simulink model "Simple_caps_working4"  (R2018b)
settings: Solver=ode5  StartTime=0.0  StopTime=10  FixedStep=Ts  RelTol=1e-3
PreLoadFcn:
  | setMatlabPaths
  | Ts = 1e-4
  | C = 100e-6
undefined symbols (not defined in the file or in its folder): DiscIntNeverNeededParam, sigbuilder_block
libraries: Simple_lib x61, peGeneralControl x3, simulink x1
settings Model: NumberOfSteps=1000  Creator=billw  LastModifiedBy=billw

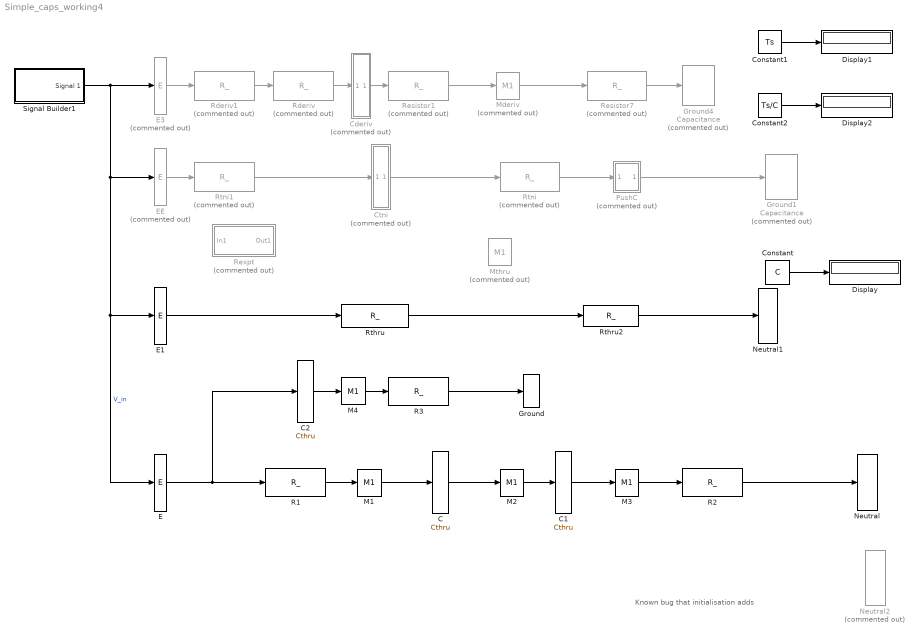
== system Simple_caps_working4 ==
  note: Known bug that initialisation adds
  C : Simple_lib/Electronics/Cthru  C=C  Q_0=0
      settings: AttributesFormatString=%<C>F
  C1 : Simple_lib/Electronics/Cthru  C=C  Q_0=0
      settings: AttributesFormatString=%<C>F
  C2 : Simple_lib/Electronics/Cthru  C=0.001  Q_0=0
      settings: AttributesFormatString=%<C>F
  "Cderiv " : Subsystem  Commented=on  mask{C=C, Q_0=0}
      mask prompts: C "Capacitance"; Q_0 "Initial Charge (C)"
      settings: AttributesFormatString=%<C>F
      mask Display:
      | %plot([1.0 1.8 1.8 1.0], [0 .1 -.1 0])
      | %patch([-1 -1 -.7 -.7 -1], [-1 1 1 -1 -1])
      | %patch([1 1 .7 .7 1], [-1 1 1 -1 -1])
      | plot([-1 -1], [-1 1])
      | plot([1 1], [-1 1])
      | color('white')
      | plot([-1.1 -1.1], [-1 1])
      | plot([1.1 1.1], [-1 1])
  Constant : Constant  Value=C
  Constant1 : Constant  Value=Ts
  Constant2 : Constant  Value=Ts/C
  Ctni : Subsystem  Commented=on  mask{C=C, Q_0=0}
      mask prompts: C "Capacitance"; Q_0 "Initial Charge (C)"
      settings: AttributesFormatString=%<C>F
      mask Display:
      | %plot([1.0 1.8 1.8 1.0], [0 .1 -.1 0])
      | %patch([-1 -1 -.7 -.7 -1], [-1 1 1 -1 -1])
      | %patch([1 1 .7 .7 1], [-1 1 1 -1 -1])
      | plot([-1 -1], [-1 1])
      | plot([1 1], [-1 1])
      | color('white')
      | plot([-1.1 -1.1], [-1 1])
      | plot([1.1 1.1], [-1 1])
  Display : Display
  Display1 : Display
  Display2 : Display
  E : Simple_lib/Electronics/E  Vbatt=0
      settings: AttributesFormatString=EMF: %<Vbatt> V
  E1 : Simple_lib/Electronics/E  Vbatt=0
      settings: AttributesFormatString=EMF: %<Vbatt> V
  E3 : Simple_lib/Electronics/E  Commented=on  Vbatt=0
      settings: AttributesFormatString=EMF: %<Vbatt> V
  EE : Simple_lib/Electronics/E  Commented=on  Vbatt=0
      settings: AttributesFormatString=EMF: %<Vbatt> V
  Ground : Simple_lib/Electronics/Ground  SystemSampleTime=-1
      link override Rgnd: R=1
  Ground1 : Simple_lib/Electronics/Capacitance  Commented=on  C=inf  V0=0
      settings: AttributesFormatString=%<C> F
  Ground4 : Simple_lib/Electronics/Capacitance  Commented=on  C=inf  V0=0
      settings: AttributesFormatString=%<C> F
  M{1..4} (4 alike) : Simple_lib/Electronics/M1  SystemSampleTime=-1
  Mderiv : Simple_lib/Electronics/M1  Commented=on  SystemSampleTime=-1
  Mthru : Simple_lib/Electronics/M1  Commented=on  SystemSampleTime=-1
  Neutral : Simple_lib/Electronics/Neutral  V0=0
      settings: AttributesFormatString=%<V0> V
  Neutral1 : Simple_lib/Electronics/Neutral  V0=-10
      settings: AttributesFormatString=%<V0> V
  Neutral2 : Simple_lib/Electronics/Neutral  Commented=on  V0=-9
      settings: AttributesFormatString=%<V0> V
  PushC : Subsystem  Commented=on  mask{C=C}
      mask prompts: C "Capacitance (Farads)"
      mask Display:
      | plot([-1 -.9 -.5 0 .5 .9 1  .9  .5  0 -.5 -.9 -1],      [ 0  .5 .9 1 .9 .5 0 -.5 -.9 -1 -.9 -.5  0]);
      | disp('M')
  R1 : Simple_lib/Electronics/R_  Exponent=3  R=1000
      settings: AttributesFormatString=%<R> Ohm
  R2 : Simple_lib/Electronics/R_  Exponent=3  R=1000
      link override at: slew_rate=inf
      settings: AttributesFormatString=%<R> Ohm
  R3 : Simple_lib/Electronics/R_  Exponent=3  R=1000
      settings: AttributesFormatString=%<R> Ohm
  Rderiv : Simple_lib/Electronics/R_  Commented=on  Exponent=0  R=1
      settings: AttributesFormatString=%<R> Ohm
  Rderiv1 : Simple_lib/Electronics/R_  Commented=on  Exponent=0  R=1
      settings: AttributesFormatString=%<R> Ohm
  Resistor1 : Simple_lib/Electronics/R_  Commented=on  Exponent=0  R=1
      link override at: slew_rate=inf
      link override at/Saturation1: LowerLimit=1e-24
      link override thru/1//R1: Gain=-1
      settings: AttributesFormatString=%<R> Ohm
  Resistor7 : Simple_lib/Electronics/R_  Commented=on  Exponent=0  R=1
      link override at: slew_rate=inf
      link override at/Saturation1: LowerLimit=1e-24
      link override thru/1//R1: Gain=-1
      settings: AttributesFormatString=%<R> Ohm
  Rexpt : Subsystem  Commented=on  AncestorBlock=Simple_lib/Electronics/R_  mask(Circuit Resistor){Mantissa=1.0, Exponent=0, R=1}
      mask prompts: Mantissa "Resistance (Ohm)"; Exponent "e"
      mask help: This block contains an Ohmic Resistance, and a test point at its outport.
      mask init:
      | newR = str2num(Mantissa) * 10^Exponent;
      | set(gcbh,'R', num2str(newR))
      settings: AttributesFormatString=%<R> Ohm
      mask Help:
      | Choose one of the standard resistance values or type your own.
      | e means the power of 10 that the chosen resistance value will be multiplied by to make the actual resistance used.
      mask TypeOptions Mantissa: 1.0 | 1.2 | 1.5 | 1.8 | 2.2 | 2.7 | 3.3 | 3.9 | 4.7 | 5.6 | 6.8 | 8.2
      mask DialogControl Exponent Tooltip: Times this power of ten
      mask Display:
      | %color('black')
      | %plot([1.0 1.18 1.18 1.0], [0 .2 -.2 0])
      | plot([-8:8]/8, [0 1 0 -1 0 1 0 -1 0 1 0 -1 0 1 0 -1 0])
      | 
      | color('white')
      | plot([-1 1 1 -1 -1], [-1 -1 1 1 -1])
  Rthru : Simple_lib/Electronics/R_  Exponent=3  R=1000
      settings: AttributesFormatString=%<R> Ohm
  Rthru2 : Simple_lib/Electronics/R_  Exponent=3  R=1000
      settings: AttributesFormatString=%<R> Ohm
  Rtni : Simple_lib/Electronics/R_  Commented=on  Exponent=0  R=1
      settings: AttributesFormatString=%<R> Ohm
  Rtni1 : Simple_lib/Electronics/R_  Commented=on  Exponent=0  R=1
      settings: AttributesFormatString=%<R> Ohm
  Signal Builder1 : Subsystem  Tag=STV Subsys  LoadFcn=sigbuilder_block('load');  StartFcn=sigbuilder_block('start');  StopFcn=sigbuilder_block('stop');  ClipboardFcn=sigbuilder_block('clipboard');  mask(Sigbuilder block){tuvar=[0:10]}
      mask help: Simulink:masks:SigbuilderBlock_MD
      mask init:
      | if ~strcmp(get_param(bdroot(gcbh),'SimulationStatus'),'stopped') tuvar = sigbuilder_block('maskInit'); end
      settings: CopyFcn=sigbuilder_block('copy');  DeleteFcn=sigbuilder_block('delete');  ModelCloseFcn=sigbuilder_block('modelClose');  PreSaveFcn=sigbuilder_block('preSave');  PauseFcn=sigbuilder_block('pause');  ContinueFcn=sigbuilder_block('continue');  NameChangeFcn=sigbuilder_block('namechange');  OpenFcn=sigbuilder_block('open',[601.8 232.8 544.8 353.4 ]);  CloseFcn=sigbuilder_block('close');
      mask Display: plot(0, 0, 100, 100,[2, 2, 32, 32, 2], [68, 8, 8, 68, 68],[32, 2], [38, 38], [32, 19, 2],[53, 60, 44], [32, 17, 17, 2],[16, 16, 31, 31]);txt = getActiveGroup(gcbh);text(2, 100, txt,'verticalAlignment', 'top');
  wires:
  PushC/1(Out1) -> Ground1/1
  EE/1 -> Rtni1/1
  Rtni/1 -> PushC/1(In1)
  Mderiv/1 -> Resistor7/1
  E3/1 -> Rderiv1/1
  Rderiv/1 -> "Cderiv "/1(In1)
  "Cderiv "/1(Out1) -> Resistor1/1
  E1/1 -> Rthru/1
  Rthru/1 -> Rthru2/1
  Resistor1/1 -> Mderiv/1
  Resistor7/1 -> Ground4/1
  Rtni1/1 -> Ctni/1(In1)
  Rderiv1/1 -> Rderiv/1
  Ctni/1(Out1) -> Rtni/1
  Constant/1 -> Display/1
  Constant2/1 -> Display2/1
  Constant1/1 -> Display1/1
  Rthru2/1 -> Neutral1/1
  Signal Builder1/1(Signal 1) -> E/1, E1/1, EE/1, E3/1  "V_in"
  R1/1 -> M1/1
  M1/1 -> C/1
  E/1 -> C2/1, R1/1
  C/1 -> M2/1
  M2/1 -> C1/1
  R2/1 -> Neutral/1
  C1/1 -> M3/1
  M3/1 -> R2/1
  C2/1 -> M4/1
  R3/1 -> Ground/1
  M4/1 -> R3/1

== system Simple_caps_working4/Cderiv  ==
  In1 : Inport
  C2 : Subsystem  Commented=on  AncestorBlock=Simple_lib/Electronics/C1  mask{C=1e-3}
      mask prompts: C "Capacitance"
      settings: AttributesFormatString=%<C> F
      mask Display:
      | plot([-1 1], [0.5 0.5])
      | plot([-1 1], [-0.5 -0.5])
      | 
      | 
      | color('white')
      | plot([-1 1 1 -1 -1], [-1 -1 1 1 -1])
  C3 : Subsystem  AncestorBlock=Simple_lib/Electronics/C1  mask{C=1e-3}
      mask prompts: C "Capacitance"
      settings: AttributesFormatString=%<C> F
      mask Display:
      | plot([-1 1], [0.5 0.5])
      | plot([-1 1], [-0.5 -0.5])
      | 
      | 
      | color('white')
      | plot([-1 1 1 -1 -1], [-1 -1 1 1 -1])
  Cap : Subsystem  Commented=on  AncestorBlock=Simple_lib/Electronics/C1  mask{C=C}
      mask prompts: C "Capacitance"
      settings: AttributesFormatString=%<C> F
      mask Display:
      | plot([-1 1], [0.5 0.5])
      | plot([-1 1], [-0.5 -0.5])
      | 
      | 
      | color('white')
      | plot([-1 1 1 -1 -1], [-1 -1 1 1 -1])
  Cgood : Subsystem  AncestorBlock=Simple_lib/Electronics/C1  mask{C=10e-6}
      mask prompts: C "Capacitance"
      settings: AttributesFormatString=%<C> F
      mask Display:
      | plot([-1 1], [0.5 0.5])
      | plot([-1 1], [-0.5 -0.5])
      | 
      | 
      | color('white')
      | plot([-1 1 1 -1 -1], [-1 -1 1 1 -1])
  from : Simple_lib/Electronics/TP  V_0=0.0  C=0  conserved_quantity_name=Q  energy_name=E
  Out1 : Outport
  wires:
  In1/1 -> C3/2(neg)
  from/1 -> C3/1(pos), Out1/1

== system Simple_caps_working4/Ctni ==
  In1 : Inport
  C2 : Subsystem  Commented=on  AncestorBlock=Simple_lib/Electronics/C1  mask{C=1e-3}
      mask prompts: C "Capacitance"
      settings: AttributesFormatString=%<C> F
      mask Display:
      | plot([-1 1], [0.5 0.5])
      | plot([-1 1], [-0.5 -0.5])
      | 
      | 
      | color('white')
      | plot([-1 1 1 -1 -1], [-1 -1 1 1 -1])
  C3 : Subsystem  AncestorBlock=Simple_lib/Electronics/C1  mask{C=1e-3}
      mask prompts: C "Capacitance"
      settings: AttributesFormatString=%<C> F
      mask Display:
      | plot([-1 1], [0.5 0.5])
      | plot([-1 1], [-0.5 -0.5])
      | 
      | 
      | color('white')
      | plot([-1 1 1 -1 -1], [-1 -1 1 1 -1])
  Cap : Subsystem  Commented=on  AncestorBlock=Simple_lib/Electronics/C1  mask{C=C}
      mask prompts: C "Capacitance"
      settings: AttributesFormatString=%<C> F
      mask Display:
      | plot([-1 1], [0.5 0.5])
      | plot([-1 1], [-0.5 -0.5])
      | 
      | 
      | color('white')
      | plot([-1 1 1 -1 -1], [-1 -1 1 1 -1])
  Cgood : Subsystem  AncestorBlock=Simple_lib/Electronics/C1  mask{C=10e-6}
      mask prompts: C "Capacitance"
      settings: AttributesFormatString=%<C> F
      mask Display:
      | plot([-1 1], [0.5 0.5])
      | plot([-1 1], [-0.5 -0.5])
      | 
      | 
      | color('white')
      | plot([-1 1 1 -1 -1], [-1 -1 1 1 -1])
  from : Simple_lib/Electronics/TP  V_0=0.0  C=0  conserved_quantity_name=Q  energy_name=E
  Out1 : Outport
  wires:
  In1/1 -> C3/2(neg)
  from/1 -> C3/1(pos), Out1/1

== system Simple_caps_working4/PushC ==
  In1 : Inport
  SeriesCapacitance : Subsystem
  _at : Simple_lib/Electronics/_out  Tag=Electrical  Level=V  Flow=I
  _thru : Subsystem  AncestorBlock=Simple_lib/Electronics/_in  InitFcn=""  mask{Level=V, Flow=I}
      mask prompts: Level "Level variable name:"; Flow "Flow variable name:"
      mask init:
      | init_in
      mask Display:
      | %% Icon for flow in
      | % Signally design
      | %plot([0 2 2 3], [1 1 0 0])
      | %plot([1 3 2 1 0 2], [0.6 0.6 0.4 0.6 0.4 0.4])
      | %patch([1 3 2],[0.6 0.6 0.4])
      | %plot([0 1 1], [1 1 0.6])
      | %plot([1 1 0], [0.4 -1 -1])
      | 
      | %color('white')
      | %plot([0 3], [2 2])
      | %plot([0 3], [-2 -2])
      | 
      | %% Bolder design
      | %patch( [0 1 -1], [0 1 1])
      | %plot( [-1 1], [1.05 1.05])
      | %patch( [-0.1 -0.1 -1], [0.95 0 0.95])
      | patch( [-0.1 -0.1 -1], [1 0 1])
      | patch( [0.1 0.1 1], [1 0 1])
      | plot( [0.1 1 -1 -0.1], [0 -2 -2 0]*0.5)
      | %patch( [-0.1 0.1 0.1 -0.1], [0 0 1 1], [1 1 1])
      | %patch( [-1 0.1 0.1 -1], [1 1 0.95 0.95], [1 1 1])
      | 
      | %% Size the box
      | color('white')
      | plot( [-1 1], [2 2])
      | plot( [-1 1], -[2 2])
  Out1 : Outport
  wires:
  In1/1 -> _thru/1(in)
  _at/1 -> Out1/1
  _thru/1(out) -> _at/1
  _at/2 -> SeriesCapacitance/1(In1)
  SeriesCapacitance/1(Out1) -> _thru/2(back)

== system Simple_caps_working4/Rexpt ==
  In1 : Inport
  Math Function : Math  Operator=reciprocal  SaturateOnIntegerOverflow=on
  R1 : Simple_lib/Electronics/R1  Commented=on  R=R
      settings: AttributesFormatString=%<R> Ohms
  Sine Wave : Sin  Amplitude=.1  Bias=.2  SampleTime=0
  VR : Simple_lib/Electronics/VR  SystemSampleTime=-1
  at : Subsystem  AncestorBlock=Simple_lib/Electronics/TP  mask{V_0=20, slew_rate=1000, conserved_quantity_name=Q, energy_name=E}
      mask prompts: V_0 "Iniitial Potential (V)"; slew_rate "Max +/- slew rate (V/s)"; conserved_quantity_name "Conserved quantity name"; energy_name "Energy name"
      mask init:
      | init_lump
      mask Display:
      | plot([-1 -.9 -.5 0 .5 .9 1  .9  .5  0 -.5 -.9 -1],      [ 0  .5 .9 1 .9 .5 0 -.5 -.9 -1 -.9 -.5  0]);
      | %disp(get(gcbh,'Name'))
  Out1 : Outport
  wires:
  at/1(out) -> VR/3, Out1/1
  In1/1 -> VR/1
  Sine Wave/1 -> Math Function/1  "R"
  Math Function/1 -> VR/2  "G"

== system Simple_caps_working4/Signal Builder1 ==
  Demux : Demux  Tag=STV Demux  Outputs=1
  FromWs : FromWorkspace  Tag=STV FromWs  VariableName=tuvar  SampleTime=0
      SigBuilderData=|
      | common.afterFinalStr = 'Extrapolate'
      | common.sampleTime = 0
      | dataSet.timeRange = [0 10]
      | dataSet.name = 'Group 1'
      | sbobj.Groups.Name = 'Group 1'
      | sbobj.Groups.Signals.Name = 'Signal 1'
      | sbobj.Groups.Signals.XData = [0 2.98 2.98 4 4 6 6 10]
      | sbobj.Groups.Signals.YData = [0.39 0.39 0.5 0.5 1 1 0.225 0.225]
  Signal 1 : Outport  Tag=STV Outport
  wires:
  FromWs/1 -> Demux/1
  Demux/1 -> Signal 1/1

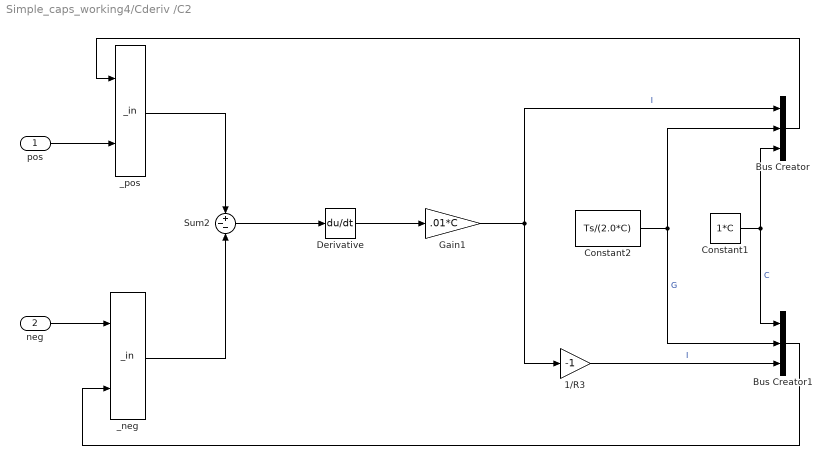
== system Simple_caps_working4/Cderiv /C2 ==
  pos : Inport
  neg : Inport  Port=2
  1/R3 : Gain  Gain=-1
  Bus Creator : BusCreator  Inputs=3
  Bus Creator1 : BusCreator  Inputs=3
  Constant1 : Constant  Value=1*C
  Constant2 : Constant  Value=Ts/(2.0*C)
  Derivative : Derivative
  Gain1 : Gain  Gain=.01*C
  Sum2 : Sum  Inputs=+--
  _neg : Simple_lib/Electronics/_in  Level=V  Flow=I
  _pos : Simple_lib/Electronics/_in  Level=V  Flow=I
  wires:
  Constant1/1 -> Bus Creator/3, Bus Creator1/1  "C"
  Constant2/1 -> Bus Creator/2, Bus Creator1/2  "G"
  1/R3/1 -> Bus Creator1/3  "I"
  Sum2/1 -> Derivative/1
  _neg/1 -> Sum2/3
  Bus Creator1/1 -> _neg/2
  Bus Creator/1 -> _pos/2
  _pos/1 -> Sum2/1
  pos/1 -> _pos/1
  neg/1 -> _neg/1
  Derivative/1 -> Gain1/1
  Gain1/1 -> 1/R3/1, Bus Creator/1  "I"

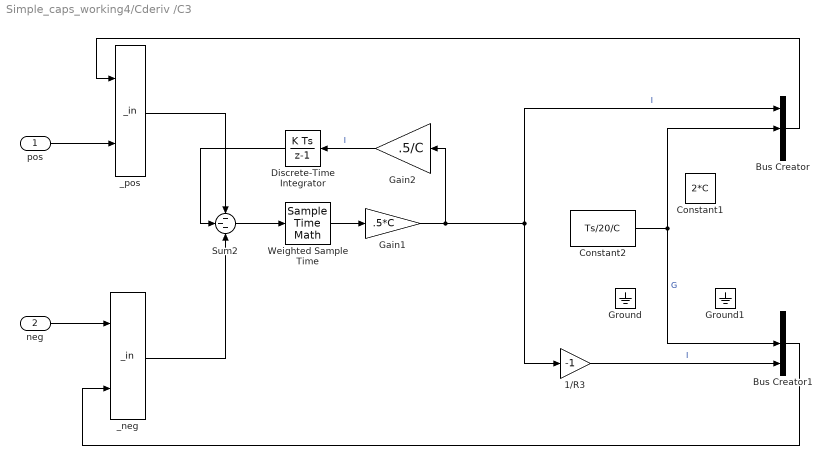
== system Simple_caps_working4/Cderiv /C3 ==
  pos : Inport
  neg : Inport  Port=2
  1/R3 : Gain  Gain=-1
  Bus Creator : BusCreator  Inputs=3
  Bus Creator1 : BusCreator  Inputs=3
  Constant1 : Constant  Value=2*C
  Constant2 : Constant  Value=Ts/20/C
  Discrete-Time Integrator : DiscreteIntegrator  SampleTime=-1  ICPrevOutput=DiscIntNeverNeededParam  ICPrevScaledInput=DiscIntNeverNeededParam
  Gain1 : Gain  Gain=.5*C
  Gain2 : Gain  Gain=.5/C
  Ground : Ground
  Ground1 : Ground
  Sum2 : Sum  Inputs=---
  Weighted Sample Time : SampleTimeMath  TsampMathOp=/  weightValue=1.1
  _neg : Simple_lib/Electronics/_in  Level=V  Flow=I
  _pos : Simple_lib/Electronics/_in  Level=V  Flow=I
  wires:
  ? -> Bus Creator/3, Bus Creator1/1  "C"
  Constant2/1 -> Bus Creator/2, Bus Creator1/2  "G"
  1/R3/1 -> Bus Creator1/3  "I"
  Sum2/1 -> Weighted Sample Time/1
  _neg/1 -> Sum2/3
  Bus Creator1/1 -> _neg/2
  Bus Creator/1 -> _pos/2
  _pos/1 -> Sum2/1
  pos/1 -> _pos/1
  neg/1 -> _neg/1
  Weighted Sample Time/1 -> Gain1/1
  Gain1/1 -> 1/R3/1, Bus Creator/1, Gain2/1  "I"
  Discrete-Time Integrator/1 -> Sum2/2
  Gain2/1 -> Discrete-Time Integrator/1  "I"

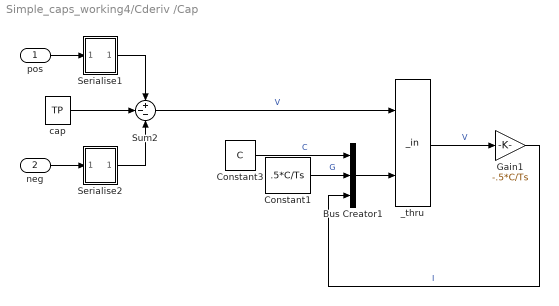
== system Simple_caps_working4/Cderiv /Cap ==
  pos : Inport
  neg : Inport  Port=2
  Bus Creator1 : BusCreator  Inputs=3
  Constant1 : Constant  Value=.5*C/Ts
  Constant3 : Constant  Value=C
  Gain1 : Gain  Gain=-.5*C/Ts
  Serialise1 : Subsystem
      mask Display:
      | plot([-1 -.9 -.5 0 .5 .9 1  .9  .5  0 -.5 -.9 -1],      [ 0  .5 .9 1 .9 .5 0 -.5 -.9 -1 -.9 -.5  0]);
      | disp('M')
  Serialise2 : Subsystem
      mask Display:
      | plot([-1 -.9 -.5 0 .5 .9 1  .9  .5  0 -.5 -.9 -1],      [ 0  .5 .9 1 .9 .5 0 -.5 -.9 -1 -.9 -.5  0]);
      | disp('M')
  Sum2 : Sum  Inputs=+--
  _thru : Simple_lib/Electronics/_in  Level=V  Flow=I
  cap : Simple_lib/Electronics/TP  V_0=0.0  C=0  conserved_quantity_name=Q  energy_name=E
      link override Saturation1: LowerLimit=0
  wires:
  pos/1 -> Serialise1/1(In1)
  Bus Creator1/1 -> _thru/2
  neg/1 -> Serialise2/1(In1)
  Constant1/1 -> Bus Creator1/2  "G"
  Constant3/1 -> Bus Creator1/1  "C"
  Gain1/1 -> Bus Creator1/3  "I"
  _thru/1 -> Gain1/1  "V"
  Sum2/1 -> _thru/1  "V"
  Serialise1/1(Out1) -> Sum2/1
  Serialise2/1(Out1) -> Sum2/3
  cap/1 -> Sum2/2

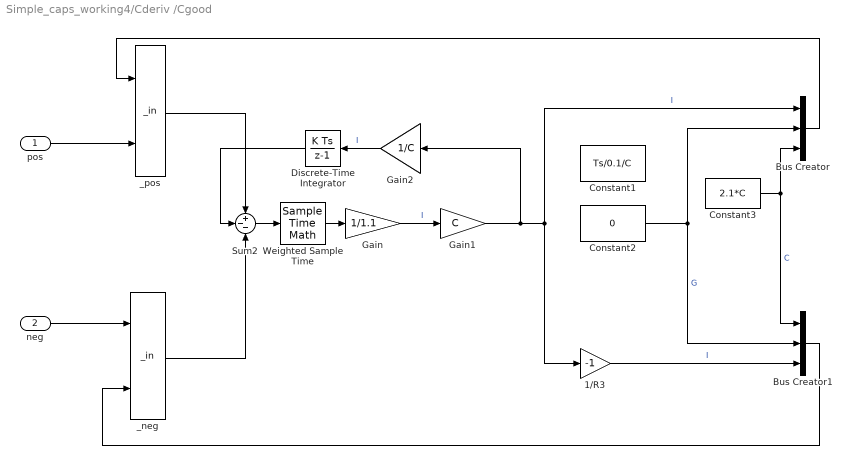
== system Simple_caps_working4/Cderiv /Cgood ==
  pos : Inport
  neg : Inport  Port=2
  1/R3 : Gain  Gain=-1
  Bus Creator : BusCreator  Inputs=3
  Bus Creator1 : BusCreator  Inputs=3
  Constant1 : Constant  Value=Ts/0.1/C
  Constant2 : Constant  Value=0
  Constant3 : Constant  Value=2.1*C
  Discrete-Time Integrator : DiscreteIntegrator  SampleTime=-1  ICPrevOutput=DiscIntNeverNeededParam  ICPrevScaledInput=DiscIntNeverNeededParam
  Gain : Gain  Gain=1/1.1
  Gain1 : Gain  Gain=C
  Gain2 : Gain  Gain=1/C
  Sum2 : Sum  Inputs=+--
  Weighted Sample Time : SampleTimeMath  TsampMathOp=/  weightValue=1
  _neg : Simple_lib/Electronics/_in  Level=V  Flow=I
  _pos : Simple_lib/Electronics/_in  Level=V  Flow=I
  wires:
  Gain2/1 -> Discrete-Time Integrator/1  "I"
  Discrete-Time Integrator/1 -> Sum2/2
  Gain/1 -> Gain1/1  "I"
  Weighted Sample Time/1 -> Gain/1
  _pos/1 -> Sum2/1
  Bus Creator/1 -> _pos/2
  Bus Creator1/1 -> _neg/2
  _neg/1 -> Sum2/3
  Sum2/1 -> Weighted Sample Time/1
  1/R3/1 -> Bus Creator1/3  "I"
  Constant2/1 -> Bus Creator1/2, Bus Creator/2  "G"
  Constant3/1 -> Bus Creator1/1, Bus Creator/3  "C"
  pos/1 -> _pos/1
  neg/1 -> _neg/1
  Gain1/1 -> Gain2/1, Bus Creator/1, 1/R3/1  "I"

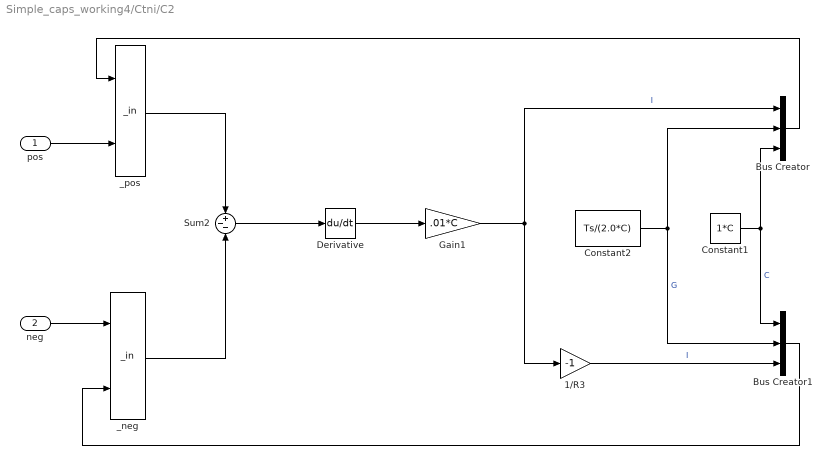
== system Simple_caps_working4/Ctni/C2 ==
  pos : Inport
  neg : Inport  Port=2
  1/R3 : Gain  Gain=-1
  Bus Creator : BusCreator  Inputs=3
  Bus Creator1 : BusCreator  Inputs=3
  Constant1 : Constant  Value=1*C
  Constant2 : Constant  Value=Ts/(2.0*C)
  Derivative : Derivative
  Gain1 : Gain  Gain=.01*C
  Sum2 : Sum  Inputs=+--
  _neg : Simple_lib/Electronics/_in  Level=V  Flow=I
  _pos : Simple_lib/Electronics/_in  Level=V  Flow=I
  wires:
  Constant1/1 -> Bus Creator/3, Bus Creator1/1  "C"
  Constant2/1 -> Bus Creator/2, Bus Creator1/2  "G"
  1/R3/1 -> Bus Creator1/3  "I"
  Sum2/1 -> Derivative/1
  _neg/1 -> Sum2/3
  Bus Creator1/1 -> _neg/2
  Bus Creator/1 -> _pos/2
  _pos/1 -> Sum2/1
  pos/1 -> _pos/1
  neg/1 -> _neg/1
  Derivative/1 -> Gain1/1
  Gain1/1 -> 1/R3/1, Bus Creator/1  "I"

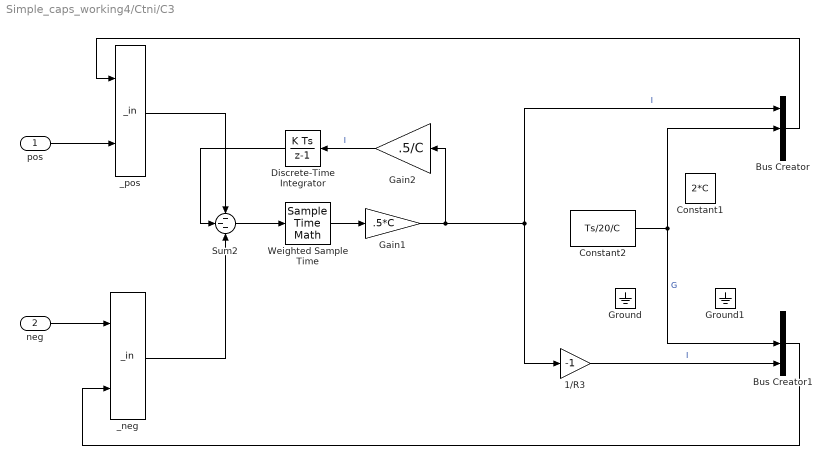
== system Simple_caps_working4/Ctni/C3 ==
  pos : Inport
  neg : Inport  Port=2
  1/R3 : Gain  Gain=-1
  Bus Creator : BusCreator  Inputs=3
  Bus Creator1 : BusCreator  Inputs=3
  Constant1 : Constant  Value=2*C
  Constant2 : Constant  Value=Ts/20/C
  Discrete-Time Integrator : DiscreteIntegrator  SampleTime=-1  ICPrevOutput=DiscIntNeverNeededParam  ICPrevScaledInput=DiscIntNeverNeededParam
  Gain1 : Gain  Gain=.5*C
  Gain2 : Gain  Gain=.5/C
  Ground : Ground
  Ground1 : Ground
  Sum2 : Sum  Inputs=---
  Weighted Sample Time : SampleTimeMath  TsampMathOp=/  weightValue=1.1
  _neg : Simple_lib/Electronics/_in  Level=V  Flow=I
  _pos : Simple_lib/Electronics/_in  Level=V  Flow=I
  wires:
  ? -> Bus Creator/3, Bus Creator1/1  "C"
  Constant2/1 -> Bus Creator/2, Bus Creator1/2  "G"
  1/R3/1 -> Bus Creator1/3  "I"
  Sum2/1 -> Weighted Sample Time/1
  _neg/1 -> Sum2/3
  Bus Creator1/1 -> _neg/2
  Bus Creator/1 -> _pos/2
  _pos/1 -> Sum2/1
  pos/1 -> _pos/1
  neg/1 -> _neg/1
  Weighted Sample Time/1 -> Gain1/1
  Gain1/1 -> 1/R3/1, Bus Creator/1, Gain2/1  "I"
  Discrete-Time Integrator/1 -> Sum2/2
  Gain2/1 -> Discrete-Time Integrator/1  "I"

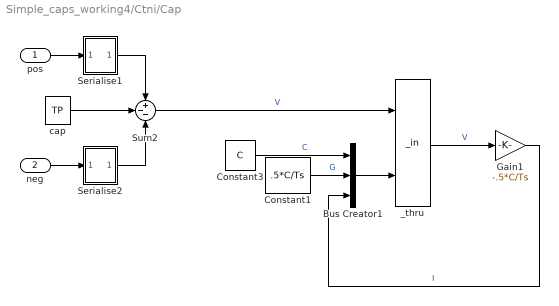
== system Simple_caps_working4/Ctni/Cap ==
  pos : Inport
  neg : Inport  Port=2
  Bus Creator1 : BusCreator  Inputs=3
  Constant1 : Constant  Value=.5*C/Ts
  Constant3 : Constant  Value=C
  Gain1 : Gain  Gain=-.5*C/Ts
  Serialise1 : Subsystem
      mask Display:
      | plot([-1 -.9 -.5 0 .5 .9 1  .9  .5  0 -.5 -.9 -1],      [ 0  .5 .9 1 .9 .5 0 -.5 -.9 -1 -.9 -.5  0]);
      | disp('M')
  Serialise2 : Subsystem
      mask Display:
      | plot([-1 -.9 -.5 0 .5 .9 1  .9  .5  0 -.5 -.9 -1],      [ 0  .5 .9 1 .9 .5 0 -.5 -.9 -1 -.9 -.5  0]);
      | disp('M')
  Sum2 : Sum  Inputs=+--
  _thru : Simple_lib/Electronics/_in  Level=V  Flow=I
  cap : Simple_lib/Electronics/TP  V_0=0.0  C=0  conserved_quantity_name=Q  energy_name=E
      link override Saturation1: LowerLimit=0
  wires:
  pos/1 -> Serialise1/1(In1)
  Bus Creator1/1 -> _thru/2
  neg/1 -> Serialise2/1(In1)
  Constant1/1 -> Bus Creator1/2  "G"
  Constant3/1 -> Bus Creator1/1  "C"
  Gain1/1 -> Bus Creator1/3  "I"
  _thru/1 -> Gain1/1  "V"
  Sum2/1 -> _thru/1  "V"
  Serialise1/1(Out1) -> Sum2/1
  Serialise2/1(Out1) -> Sum2/3
  cap/1 -> Sum2/2

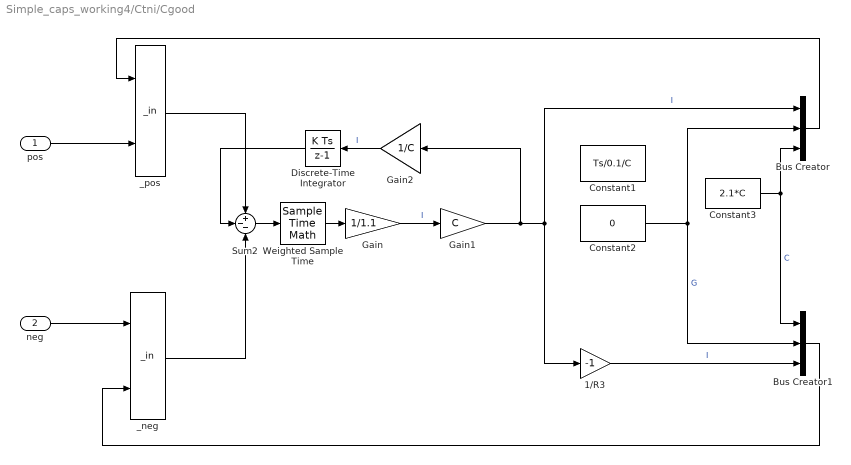
== system Simple_caps_working4/Ctni/Cgood ==
  pos : Inport
  neg : Inport  Port=2
  1/R3 : Gain  Gain=-1
  Bus Creator : BusCreator  Inputs=3
  Bus Creator1 : BusCreator  Inputs=3
  Constant1 : Constant  Value=Ts/0.1/C
  Constant2 : Constant  Value=0
  Constant3 : Constant  Value=2.1*C
  Discrete-Time Integrator : DiscreteIntegrator  SampleTime=-1  ICPrevOutput=DiscIntNeverNeededParam  ICPrevScaledInput=DiscIntNeverNeededParam
  Gain : Gain  Gain=1/1.1
  Gain1 : Gain  Gain=C
  Gain2 : Gain  Gain=1/C
  Sum2 : Sum  Inputs=+--
  Weighted Sample Time : SampleTimeMath  TsampMathOp=/  weightValue=1
  _neg : Simple_lib/Electronics/_in  Level=V  Flow=I
  _pos : Simple_lib/Electronics/_in  Level=V  Flow=I
  wires:
  Gain2/1 -> Discrete-Time Integrator/1  "I"
  Discrete-Time Integrator/1 -> Sum2/2
  Gain/1 -> Gain1/1  "I"
  Weighted Sample Time/1 -> Gain/1
  _pos/1 -> Sum2/1
  Bus Creator/1 -> _pos/2
  Bus Creator1/1 -> _neg/2
  _neg/1 -> Sum2/3
  Sum2/1 -> Weighted Sample Time/1
  1/R3/1 -> Bus Creator1/3  "I"
  Constant2/1 -> Bus Creator1/2, Bus Creator/2  "G"
  Constant3/1 -> Bus Creator1/1, Bus Creator/3  "C"
  pos/1 -> _pos/1
  neg/1 -> _neg/1
  Gain1/1 -> Gain2/1, Bus Creator/1, 1/R3/1  "I"

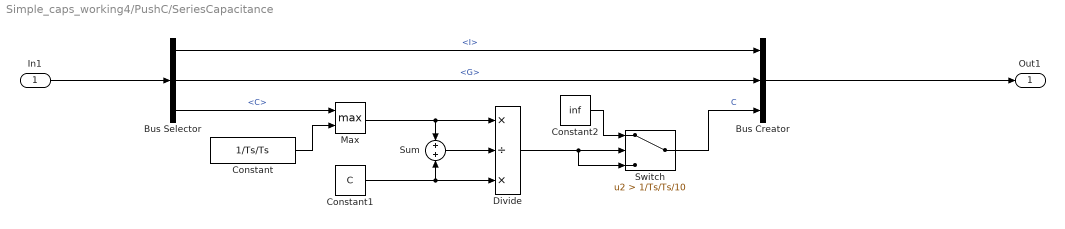
== system Simple_caps_working4/PushC/SeriesCapacitance ==
  In1 : Inport
  Bus Creator : BusCreator  Inputs=3
  Bus Selector : BusSelector  OutputSignals=I,G,C
  Constant : Constant  Value=1/Ts/Ts
  Constant1 : Constant  Value=C
  Constant2 : Constant  Value=inf
  Divide : Product  Inputs=*/*
  Max : MinMax  Function=max  Inputs=2
  Sum : Sum  Inputs=+|+
  Switch : Switch  Criteria=u2 > Threshold  Threshold=1/Ts/Ts/10
  Out1 : Outport
  wires:
  Bus Selector/2 -> Bus Creator/2  "<G>"
  Bus Selector/1 -> Bus Creator/1  "<I>"
  Bus Creator/1 -> Out1/1
  Bus Selector/3 -> Max/1  "<C>"
  In1/1 -> Bus Selector/1
  Constant/1 -> Max/2
  Max/1 -> Sum/1, Divide/1
  Constant1/1 -> Sum/2, Divide/3
  Sum/1 -> Divide/2
  Divide/1 -> Switch/3, Switch/2
  Switch/1 -> Bus Creator/3  "C"
  Constant2/1 -> Switch/1

== system Simple_caps_working4/PushC/_thru ==
  note: {\bf\_in - wraps up the {\itInflow} block}
      |
      | The init function {\itinit\_in} sets up the logging of the level and flow names.
  in : Inport
  back : Inport  Port=2
  Bus Selector : BusSelector  OutputSignals=I,G,C
  Constant : Constant  Value=[0,0,0]
  Constant1 : Constant  Value=C
  Inflow : Simple_lib/Utility/Inflow  SystemSampleTime=-1
  Mux : Mux  Inputs=3
  Sum : Sum  Inputs=|++
  Terminator : Terminator
  out : Outport
  wires:
  Mux/1 -> Sum/1
  Inflow/1 -> out/1
  Bus Selector/1 -> Mux/1  "<I>"
  Bus Selector/3 -> Terminator/1  "<C>"
  back/1 -> Bus Selector/1
  in/1 -> Inflow/1  "V"
  Bus Selector/2 -> Mux/2  "<G>"
  Sum/1 -> Inflow/2
  Constant/1 -> Sum/2
  Constant1/1 -> Mux/3

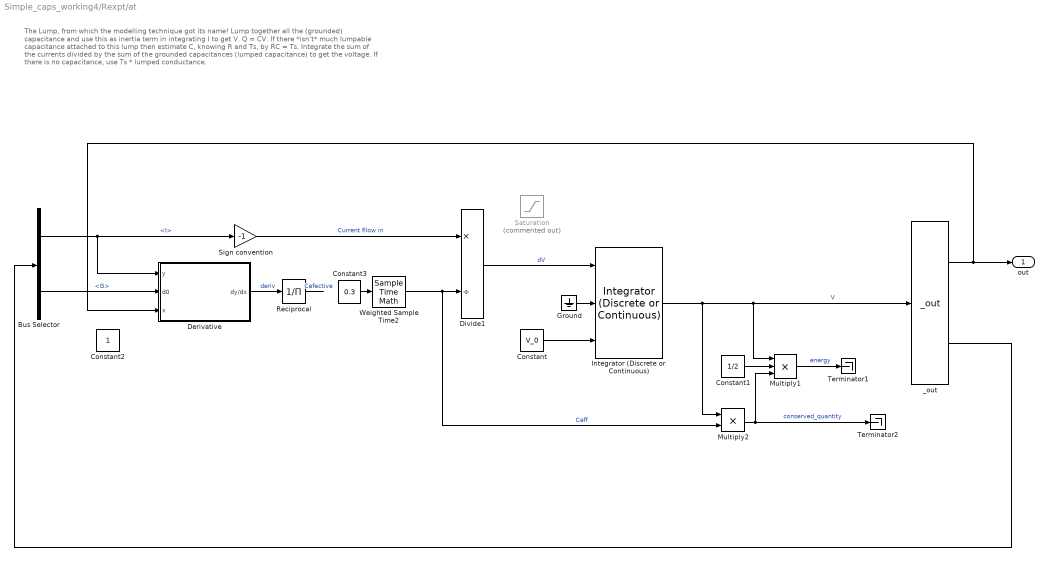
== system Simple_caps_working4/Rexpt/at ==
  note: The Lump, from which the modelling technique got its name!
      | Lump together all the (grounded) capacitance and use this as inertia term in integrating I to get V.  Q = CV.
      | If there *isn't* much lumpable capacitance attached to this lump then estimate C, knowing R and Ts, by RC = Ts.
      | Integrate the sum of the currents divided by the sum of the grounded capacitances (lumped capacitance) to get the voltage.
      | If there is no capacitance, use Ts * lumped conductance.
  Bus Selector : BusSelector  OutputSignals=I,G
  Constant : Constant  Value=V_0
  Constant1 : Constant  Value=1/2
  Constant2 : Constant
  Constant3 : Constant  Value=0.3
  Derivative : Subsystem  AncestorBlock=Simple_lib/Utility/Derivative  mask{w=2}
      mask prompts: w "weight"
  Divide1 : Product  Inputs=*/
  Ground : Ground
  Integrator (Discrete or Continuous) : peGeneralControl/Integrator (Discrete or Continuous)  LabelModeActiveChoice=Discrete  ExternalReset=level  LimitType=Anti-windup  B=inf  A=-inf  Ts=-1
  Multiply1 : Product  Inputs=3
  Multiply2 : Product
  Reciprocal : Product  Inputs=/  SaturateOnIntegerOverflow=on  RndMeth=Zero
  Saturation : Saturate  Commented=on  UpperLimit=slew_rate  LowerLimit=-slew_rate
      settings: AttributesFormatString=|
      | %<UpperLimit>
      | %<LowerLimit>
  Sign convention : Gain  Gain=-1
  Terminator1 : Terminator
  Terminator2 : Terminator
  Weighted Sample Time2 : SampleTimeMath  TsampMathOp=*  weightValue=1
  _out : Simple_lib/Electronics/_out  Tag=Electrical  Level=V  Flow=I
  out : Outport
  wires:
  Sign convention/1 -> Divide1/1  "Current fllow in"
  Integrator (Discrete or Continuous)/1 -> _out/1, Multiply1/1, Multiply2/1  "V"
  Multiply2/1 -> Multiply1/3, Terminator2/1  "conserved_quantity"
  Multiply1/1 -> Terminator1/1  "energy"
  Constant1/1 -> Multiply1/2
  Reciprocal/1 -> ?  "Cefective"
  Bus Selector/2 -> Derivative/2(d0)  "<G>"
  Constant/1 -> Integrator (Discrete or Continuous)/3
  Ground/1 -> Integrator (Discrete or Continuous)/2
  Bus Selector/1 -> Sign convention/1, Derivative/1(y)  "<I>"
  _out/2 -> Bus Selector/1
  _out/1 -> Derivative/3(x), out/1
  Divide1/1 -> Integrator (Discrete or Continuous)/1  "dV"
  Derivative/1(dy/dx) -> Reciprocal/1  "deriv"
  Weighted Sample Time2/1 -> Divide1/2, Multiply2/2  "Ceff"
  Constant3/1 -> Weighted Sample Time2/1

== system Simple_caps_working4/Cderiv /Cap/Serialise1 ==
  In1 : Inport
  Bus Creator : BusCreator  Inputs=3
  Bus Selector : BusSelector  OutputSignals=I,G,C
  Ground : Ground
  Ground2 : Ground
  Terminator1 : Terminator
  _at : Simple_lib/Electronics/_out  Tag=Electrical  Level=V  Flow=I
  _thru : Simple_lib/Electronics/_in  Level=V  Flow=I
  Out1 : Outport
  wires:
  _at/2 -> Bus Selector/1
  _thru/1 -> _at/1
  In1/1 -> _thru/1
  _at/1 -> Out1/1
  Bus Selector/1 -> Bus Creator/1  "<I>"
  Bus Selector/2 -> Bus Creator/2  "<G>"
  Bus Selector/3 -> Terminator1/1  "<C>"
  Bus Creator/1 -> _thru/2
  Ground/1 -> Bus Creator/3  "C"

== system Simple_caps_working4/Cderiv /Cap/Serialise2 ==
  In1 : Inport
  Bus Creator : BusCreator  Inputs=3
  Bus Selector : BusSelector  OutputSignals=I,G,C
  Ground : Ground
  Terminator1 : Terminator
  _at : Simple_lib/Electronics/_out  Tag=Electrical  Level=V  Flow=I
  _thru : Simple_lib/Electronics/_in  Level=V  Flow=I
  Out1 : Outport
  wires:
  _at/2 -> Bus Selector/1
  _thru/1 -> _at/1
  In1/1 -> _thru/1
  _at/1 -> Out1/1
  Bus Selector/1 -> Bus Creator/1  "<I>"
  Bus Selector/3 -> Terminator1/1  "<C>"
  Bus Creator/1 -> _thru/2
  Bus Selector/2 -> Bus Creator/2  "<G>"
  Ground/1 -> Bus Creator/3  "C"

== system Simple_caps_working4/Ctni/Cap/Serialise1 ==
  In1 : Inport
  Bus Creator : BusCreator  Inputs=3
  Bus Selector : BusSelector  OutputSignals=I,G,C
  Ground : Ground
  Ground2 : Ground
  Terminator1 : Terminator
  _at : Simple_lib/Electronics/_out  Tag=Electrical  Level=V  Flow=I
  _thru : Simple_lib/Electronics/_in  Level=V  Flow=I
  Out1 : Outport
  wires:
  _at/2 -> Bus Selector/1
  _thru/1 -> _at/1
  In1/1 -> _thru/1
  _at/1 -> Out1/1
  Bus Selector/1 -> Bus Creator/1  "<I>"
  Bus Selector/2 -> Bus Creator/2  "<G>"
  Bus Selector/3 -> Terminator1/1  "<C>"
  Bus Creator/1 -> _thru/2
  Ground/1 -> Bus Creator/3  "C"

== system Simple_caps_working4/Ctni/Cap/Serialise2 ==
  In1 : Inport
  Bus Creator : BusCreator  Inputs=3
  Bus Selector : BusSelector  OutputSignals=I,G,C
  Ground : Ground
  Terminator1 : Terminator
  _at : Simple_lib/Electronics/_out  Tag=Electrical  Level=V  Flow=I
  _thru : Simple_lib/Electronics/_in  Level=V  Flow=I
  Out1 : Outport
  wires:
  _at/2 -> Bus Selector/1
  _thru/1 -> _at/1
  In1/1 -> _thru/1
  _at/1 -> Out1/1
  Bus Selector/1 -> Bus Creator/1  "<I>"
  Bus Selector/3 -> Terminator1/1  "<C>"
  Bus Creator/1 -> _thru/2
  Bus Selector/2 -> Bus Creator/2  "<G>"
  Ground/1 -> Bus Creator/3  "C"

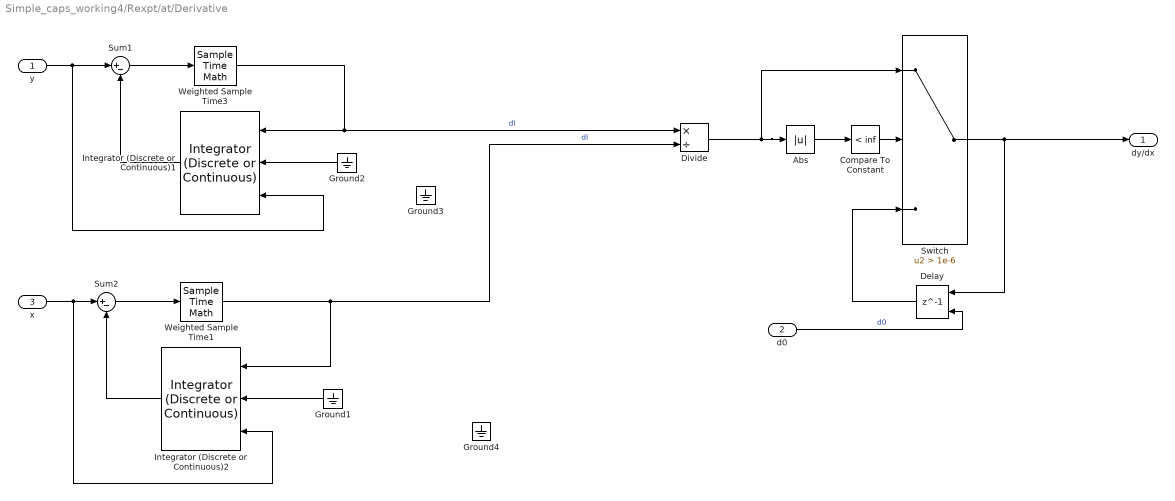
== system Simple_caps_working4/Rexpt/at/Derivative ==
  y : Inport
  d0 : Inport  Port=2
  x : Inport  Port=3
  Abs : Abs
  Compare To Constant : simulink/Logic and Bit Operations/Compare To Constant  relop=<  const=inf  OutDataTypeStr=boolean
  Delay : Delay  DelayLength=1  InitialConditionSource=Input port
      settings: InputPortMap=u0,p4
  Divide : Product  Inputs=*/
  Ground{1..4} (4 alike) : Ground
  Integrator (Discrete or Continuous)1 : peGeneralControl/Integrator (Discrete or Continuous)  LabelModeActiveChoice=Discrete  ExternalReset=level  LimitType=Anti-windup  B=inf  A=-inf  Ts=-1
  Integrator (Discrete or Continuous)2 : peGeneralControl/Integrator (Discrete or Continuous)  LabelModeActiveChoice=Discrete  ExternalReset=level  LimitType=Anti-windup  B=inf  A=-inf  Ts=-1
  Sum1 : Sum  Inputs=|+-
  Sum2 : Sum  Inputs=|+-
  Switch : Switch  Criteria=u2 > Threshold  Threshold=1e-6
  Weighted Sample Time1 : SampleTimeMath  TsampMathOp=/  weightValue=1
  Weighted Sample Time3 : SampleTimeMath  TsampMathOp=/  weightValue=w
  dy/dx : Outport
  wires:
  Ground1/1 -> Integrator (Discrete or Continuous)2/2
  Sum2/1 -> Weighted Sample Time1/1
  Integrator (Discrete or Continuous)2/1 -> Sum2/2
  Weighted Sample Time1/1 -> Integrator (Discrete or Continuous)2/1, Divide/2  "dI"
  Ground2/1 -> Integrator (Discrete or Continuous)1/2
  Sum1/1 -> Weighted Sample Time3/1
  Integrator (Discrete or Continuous)1/1 -> Sum1/2
  Weighted Sample Time3/1 -> Integrator (Discrete or Continuous)1/1, Divide/1  "dI"
  Switch/1 -> Delay/1, dy/dx/1
  Delay/1 -> Switch/3
  Divide/1 -> Switch/1, Abs/1
  Abs/1 -> Compare To Constant/1
  Compare To Constant/1 -> Switch/2
  y/1 -> Integrator (Discrete or Continuous)1/3, Sum1/1
  x/1 -> Integrator (Discrete or Continuous)2/3, Sum2/1
  d0/1 -> Delay/2  "d0"
